simulink model "ES004A_PwrUpSeq"  (R2013b)
settings: Solver=FixedStepDiscrete  SolverMode=SingleTasking  StartTime=0.0  StopTime=1  FixedStep=0.002  RelTol=1e-3
undefined symbols (not defined in the file): ELECGLBPRM_STRTUPSTCURRMEASWRMININTESTSTRT_CNT_U08, ELECGLBPRM_STRTUPSTDI_CNT_U08, ELECGLBPRM_STRTUPSTFLSMEMININSTRT_CNT_U08, ELECGLBPRM_STRTUPSTMTRDRVRININSTRT_CNT_U08, ELECGLBPRM_STRTUPSTPWRDISCNCTATESTSTRT_CNT_U08, ELECGLBPRM_STRTUPSTPWRDISCNCTBTESTSTRT_CNT_U08, ELECGLBPRM_STRTUPSTTMPLMONININTESTSTRT_CNT_U08, ELECGLBPRM_STRTUPSTWARMININCMPL_CNT_U08, PWRTURNOFFCTRLTHD_CNT_U08, sigbuilder_block
libraries: simulink x3
(part 2 of 2)

== system ES004A_PwrUpSeq/PwrUpSeq/PwrUpSeqPer1/SYSST_WRMININ/Power Disconnect Sequence B Running ==
  Action Port : ActionPort  ActionType=elseif
  Constant : Constant  Value=0  OutDataTypeStr=boolean
  CopyRight2 : Subsystem  Description=|  mask(Copyright Information){none=on}
      | Copyright info block.                                               
      |                                                                     
      | Place copyright information at the top of every subsystem in design.
      mask prompts: none "No parameters"
      mask help: Place copyright information at the top of every subsystem in design.
      mask Display:
      | NxtrConf = 'Nexteer Confidential';
      | 
      | sys = bdroot; %handle for the current model ("system")
      | first = get_param(sys,'Created');
      | first = first(end-3:end);  %year is last four digits
      | 
      | last = get_param(sys,'LastModifiedDate');
      | if isempty(last)
      |     last = datestr(now,'yyyy');
      | else
      |     last = last(end-3:end);
      | end
      | 
      | if strcmp(first,last)
      |     fprintf('%s -- Copyright %s Nexteer',NxtrConf,first)
      | else
      |     fprintf('%s -- %s%s- %s Nexteer',NxtrConf,char(169),first,last)
      | end
  ELECGLBPRM_STRTUPSTPWRDISCNCTBTESTSTRT_CNT_U08 : Constant  RequirementInfo="{'linktype_rmi_doors' '0000c463 (/ESG Group/FDD Module Requirements/EA4 Specific/ES004A_PowerUpSeq)' '#ES004A_88' 'true' 'REQ:  ES004A_88' '' } %GIDa_cccd4848_37b5_4367_80a4_6b67ce5050dc"  Value=ELECGLBPRM_STRTUPSTPWRDISCNCTBTESTSTRT_CNT_U08
  StrtUpSt : Outport
  SysStWrmIninCmpl : Outport  Port=2
  wires:
  ELECGLBPRM_STRTUPSTPWRDISCNCTBTESTSTRT_CNT_U08/1 -> StrtUpSt/1
  Constant/1 -> SysStWrmIninCmpl/1

== system ES004A_PwrUpSeq/PwrUpSeq/PwrUpSeqPer1/SYSST_WRMININ/Temporal Monitor Running ==
  Action Port : ActionPort  ActionType=elseif
  Constant : Constant  Value=0  OutDataTypeStr=boolean
  CopyRight2 : Subsystem  Description=|  mask(Copyright Information){none=on}
      | Copyright info block.                                               
      |                                                                     
      | Place copyright information at the top of every subsystem in design.
      mask prompts: none "No parameters"
      mask help: Place copyright information at the top of every subsystem in design.
      mask Display:
      | NxtrConf = 'Nexteer Confidential';
      | 
      | sys = bdroot; %handle for the current model ("system")
      | first = get_param(sys,'Created');
      | first = first(end-3:end);  %year is last four digits
      | 
      | last = get_param(sys,'LastModifiedDate');
      | if isempty(last)
      |     last = datestr(now,'yyyy');
      | else
      |     last = last(end-3:end);
      | end
      | 
      | if strcmp(first,last)
      |     fprintf('%s -- Copyright %s Nexteer',NxtrConf,first)
      | else
      |     fprintf('%s -- %s%s- %s Nexteer',NxtrConf,char(169),first,last)
      | end
  ELECGLBPRM_STRTUPSTTMPLMONININTESTSTRT_CNT_U08 : Constant  RequirementInfo="{'linktype_rmi_doors' '0000c463 (/ESG Group/FDD Module Requirements/EA4 Specific/ES004A_PowerUpSeq)' '#ES004A_87' 'true' 'REQ:  ES004A_87' '' } %GIDa_457ab7ff_7c8c_48ee_ba5e_1d2eb0aaa501"  Value=ELECGLBPRM_STRTUPSTTMPLMONININTESTSTRT_CNT_U08
  StrtUpSt : Outport
  SysStWrmIninCmpl : Outport  Port=2
  wires:
  ELECGLBPRM_STRTUPSTTMPLMONININTESTSTRT_CNT_U08/1 -> StrtUpSt/1
  Constant/1 -> SysStWrmIninCmpl/1

== system ES004A_PwrUpSeq/PwrUpSeq/PwrUpSeqPer1/SetTODHighState /CopyRight2 ==

== system ES004A_PwrUpSeq/PwrUpSeq/PwrUpSeqPer1/SetTODHighState /PwrTurnOffCtrl ==
  PwrTurnOffCtrl_ArgIn : Inport  OutDataTypeStr=boolean
  CopyRight2 : Subsystem  Description=|  mask(Copyright Information){none=on}
      | Copyright info block.                                               
      |                                                                     
      | Place copyright information at the top of every subsystem in design.
      mask prompts: none "No parameters"
      mask help: Place copyright information at the top of every subsystem in design.
      mask Display:
      | NxtrConf = 'Nexteer Confidential';
      | 
      | sys = bdroot; %handle for the current model ("system")
      | first = get_param(sys,'Created');
      | first = first(end-3:end);  %year is last four digits
      | 
      | last = get_param(sys,'LastModifiedDate');
      | if isempty(last)
      |     last = datestr(now,'yyyy');
      | else
      |     last = last(end-3:end);
      | end
      | 
      | if strcmp(first,last)
      |     fprintf('%s -- Copyright %s Nexteer',NxtrConf,first)
      | else
      |     fprintf('%s -- %s%s- %s Nexteer',NxtrConf,char(169),first,last)
      | end
  Terminator : Terminator
  wires:
  PwrTurnOffCtrl_ArgIn/1 -> Terminator/1

== system ES004A_PwrUpSeq/PwrUpSeq/PwrUpSeqPer1/SYSST_WRMININ/Current Measurement Running/CopyRight2 ==

== system ES004A_PwrUpSeq/PwrUpSeq/PwrUpSeqPer1/SYSST_WRMININ/Flash Memory Running/CopyRight2 ==

== system ES004A_PwrUpSeq/PwrUpSeq/PwrUpSeqPer1/SYSST_WRMININ/Gate Drive Running/CopyRight2 ==

== system ES004A_PwrUpSeq/PwrUpSeq/PwrUpSeqPer1/SYSST_WRMININ/If Action Subsystem6/CopyRight2 ==

== system ES004A_PwrUpSeq/PwrUpSeq/PwrUpSeqPer1/SYSST_WRMININ/Power Disconnect Sequence A Running/CopyRight2 ==

== system ES004A_PwrUpSeq/PwrUpSeq/PwrUpSeqPer1/SYSST_WRMININ/Power Disconnect Sequence B Running/CopyRight2 ==

== system ES004A_PwrUpSeq/PwrUpSeq/PwrUpSeqPer1/SYSST_WRMININ/Temporal Monitor Running/CopyRight2 ==

== system ES004A_PwrUpSeq/PwrUpSeq/PwrUpSeqPer1/SetTODHighState /PwrTurnOffCtrl/CopyRight2 ==
